simulink model "test_mdl"  (R2018a)
settings: Solver=VariableStepAuto  StartTime=0.0  StopTime=10.0  RelTol=1e-3
(part 2 of 8)

== system test_mdl/FD1_CAN_P702_GASD_MY21_DCV_V06/ABS_ESC/BrakeSnData_4 ==
  BrkTotTqRqArb_No_Cnt : Constant
  BrkTotTqRqArb_No_Cs : Constant
  BrkTot_Tq_Actl : Constant
  BrkTot_Tq_RqArb : Constant
  HsaStat_D_Actl : Constant
  VehRolComp_W_Actl : Constant
  VehVertComp_A_Actl : Constant
  bus_creator : BusCreator  Inputs=7
  port : Outport
  wires:
  bus_creator/1 -> port/1  "BrakeSnData_4"
  BrkTotTqRqArb_No_Cnt/1 -> bus_creator/1  "BrkTotTqRqArb_No_Cnt"
  BrkTotTqRqArb_No_Cs/1 -> bus_creator/2  "BrkTotTqRqArb_No_Cs"
  BrkTot_Tq_Actl/1 -> bus_creator/3  "BrkTot_Tq_Actl"
  BrkTot_Tq_RqArb/1 -> bus_creator/4  "BrkTot_Tq_RqArb"
  HsaStat_D_Actl/1 -> bus_creator/5  "HsaStat_D_Actl"
  VehRolComp_W_Actl/1 -> bus_creator/6  "VehRolComp_W_Actl"
  VehVertComp_A_Actl/1 -> bus_creator/7  "VehVertComp_A_Actl"

== system test_mdl/FD1_CAN_P702_GASD_MY21_DCV_V06/ABS_ESC/BrakeSnData_5 ==
  AwdLck_Tq_RqMn : Constant
  AwdLck_Tq_RqMx : Constant
  BrkCtrFnd_B_Stat : Constant
  DrvSte_D_Stat : Constant
  DrvSte_Tq_Rq : Constant
  EmgcyBrkLamp_D_Rq : Constant
  StopLamp_B_RqBrk : Constant
  bus_creator : BusCreator  Inputs=7
  port : Outport
  wires:
  bus_creator/1 -> port/1  "BrakeSnData_5"
  AwdLck_Tq_RqMn/1 -> bus_creator/1  "AwdLck_Tq_RqMn"
  AwdLck_Tq_RqMx/1 -> bus_creator/2  "AwdLck_Tq_RqMx"
  BrkCtrFnd_B_Stat/1 -> bus_creator/3  "BrkCtrFnd_B_Stat"
  DrvSte_D_Stat/1 -> bus_creator/4  "DrvSte_D_Stat"
  DrvSte_Tq_Rq/1 -> bus_creator/5  "DrvSte_Tq_Rq"
  EmgcyBrkLamp_D_Rq/1 -> bus_creator/6  "EmgcyBrkLamp_D_Rq"
  StopLamp_B_RqBrk/1 -> bus_creator/7  "StopLamp_B_RqBrk"

== system test_mdl/FD1_CAN_P702_GASD_MY21_DCV_V06/ABS_ESC/BrakeSnData_6 ==
  StePinOffst_An_Est : Constant
  StePinOffst_D_Stat : Constant
  StePinOffst_No_Cnt : Constant
  StePinOffst_No_Cs : Constant
  bus_creator : BusCreator  Inputs=4
  port : Outport
  wires:
  bus_creator/1 -> port/1  "BrakeSnData_6"
  StePinOffst_An_Est/1 -> bus_creator/1  "StePinOffst_An_Est"
  StePinOffst_D_Stat/1 -> bus_creator/2  "StePinOffst_D_Stat"
  StePinOffst_No_Cnt/1 -> bus_creator/3  "StePinOffst_No_Cnt"
  StePinOffst_No_Cs/1 -> bus_creator/4  "StePinOffst_No_Cs"

== system test_mdl/FD1_CAN_P702_GASD_MY21_DCV_V06/ABS_ESC/BrakeSysFeatures ==
  BrkFluidLvl_D_Stat : Constant
  LsmcBrkDecel_D_Stat : Constant
  VehStab_D_Stat : Constant
  VehVActlBrk_D_Qf : Constant
  VehVActlBrk_No_Cnt : Constant
  VehVActlBrk_No_Cs : Constant
  VehYawLin_W_Rq : Constant
  VehYawNonLin_W_Rq : Constant
  Veh_V_ActlBrk : Constant
  bus_creator : BusCreator  Inputs=9
  port : Outport
  wires:
  bus_creator/1 -> port/1  "BrakeSysFeatures"
  BrkFluidLvl_D_Stat/1 -> bus_creator/1  "BrkFluidLvl_D_Stat"
  LsmcBrkDecel_D_Stat/1 -> bus_creator/2  "LsmcBrkDecel_D_Stat"
  VehStab_D_Stat/1 -> bus_creator/3  "VehStab_D_Stat"
  VehVActlBrk_D_Qf/1 -> bus_creator/4  "VehVActlBrk_D_Qf"
  VehVActlBrk_No_Cnt/1 -> bus_creator/5  "VehVActlBrk_No_Cnt"
  VehVActlBrk_No_Cs/1 -> bus_creator/6  "VehVActlBrk_No_Cs"
  VehYawLin_W_Rq/1 -> bus_creator/7  "VehYawLin_W_Rq"
  VehYawNonLin_W_Rq/1 -> bus_creator/8  "VehYawNonLin_W_Rq"
  Veh_V_ActlBrk/1 -> bus_creator/9  "Veh_V_ActlBrk"

== system test_mdl/FD1_CAN_P702_GASD_MY21_DCV_V06/ABS_ESC/BrakeSysFeatures_2 ==
  Abs_B_Falt : Constant
  BpedMove_D_Actl : Constant
  BpedMove_No_Cnt : Constant
  BrkBstrVac_B_Rq : Constant
  BrkLamp_B_Rq : Constant
  ChimeBrk_B_Rq : Constant
  DrvAntiLckLamp_D_Rq : Constant
  DrvHdcLampInfo_D_Rq : Constant
  DrvHdcMsg_D_Rq : Constant
  DrvHdcWarnInfo_D_Rq : Constant
  DrvSlipCtlLamp_D_Rq : Constant
  DrvSlipCtlMde_D_Ind : Constant
  HILL_DESC_MC : Constant
  HdcMde_D_Actl : Constant
  HsaMde_D_Mem : Constant
  RearDiffElckrOpen_B_Rq : Constant
  RearDiffLck_Tq2_RqMx : Constant
  StabCtlBrk_B_Avail : Constant
  TCMode : Constant
  TRLR_SWAY_CONFIG_STAT : Constant
  TRLR_SWAY_EVNT_IN_PROG : Constant
  bus_creator : BusCreator  Inputs=21
  port : Outport
  wires:
  bus_creator/1 -> port/1  "BrakeSysFeatures_2"
  Abs_B_Falt/1 -> bus_creator/1  "Abs_B_Falt"
  BpedMove_D_Actl/1 -> bus_creator/2  "BpedMove_D_Actl"
  BpedMove_No_Cnt/1 -> bus_creator/3  "BpedMove_No_Cnt"
  BrkBstrVac_B_Rq/1 -> bus_creator/4  "BrkBstrVac_B_Rq"
  BrkLamp_B_Rq/1 -> bus_creator/5  "BrkLamp_B_Rq"
  ChimeBrk_B_Rq/1 -> bus_creator/6  "ChimeBrk_B_Rq"
  DrvAntiLckLamp_D_Rq/1 -> bus_creator/7  "DrvAntiLckLamp_D_Rq"
  DrvHdcLampInfo_D_Rq/1 -> bus_creator/8  "DrvHdcLampInfo_D_Rq"
  DrvHdcMsg_D_Rq/1 -> bus_creator/9  "DrvHdcMsg_D_Rq"
  DrvHdcWarnInfo_D_Rq/1 -> bus_creator/10  "DrvHdcWarnInfo_D_Rq"
  DrvSlipCtlLamp_D_Rq/1 -> bus_creator/11  "DrvSlipCtlLamp_D_Rq"
  DrvSlipCtlMde_D_Ind/1 -> bus_creator/12  "DrvSlipCtlMde_D_Ind"
  HILL_DESC_MC/1 -> bus_creator/13  "HILL_DESC_MC"
  HdcMde_D_Actl/1 -> bus_creator/14  "HdcMde_D_Actl"
  HsaMde_D_Mem/1 -> bus_creator/15  "HsaMde_D_Mem"
  RearDiffElckrOpen_B_Rq/1 -> bus_creator/16  "RearDiffElckrOpen_B_Rq"
  RearDiffLck_Tq2_RqMx/1 -> bus_creator/17  "RearDiffLck_Tq2_RqMx"
  StabCtlBrk_B_Avail/1 -> bus_creator/18  "StabCtlBrk_B_Avail"
  TCMode/1 -> bus_creator/19  "TCMode"
  TRLR_SWAY_CONFIG_STAT/1 -> bus_creator/20  "TRLR_SWAY_CONFIG_STAT"
  TRLR_SWAY_EVNT_IN_PROG/1 -> bus_creator/21  "TRLR_SWAY_EVNT_IN_PROG"

== system test_mdl/FD1_CAN_P702_GASD_MY21_DCV_V06/ABS_ESC/BrakeSysFeatures_3 ==
  AirDamUp_B_RqBrk : Constant
  ApaBrk_D_Stat : Constant
  AutoHoldMde_D_Ind : Constant
  AutoHoldMsgTxt_D_Rq : Constant
  AutoHoldSwMde_B_Ind : Constant
  BrkBstrVac_D_Stat : Constant
  CtaBrk_D_Stat : Constant
  DrvSlipCtlMdeMsg_D_Rq : Constant
  DrvSlipCtlOffLamp_D_Rq : Constant
  RbaBrk_D_Stat : Constant
  SelDrvMdeAwd_D_Rq : Constant
  SelDrvMdeChassis2_D_Rq : Constant
  SelDrvMdeChassis_D_Rq : Constant
  TrailCtlMsgTxt_D_Rq : Constant
  TrailCtl_D_Stat : Constant
  bus_creator : BusCreator  Inputs=15
  port : Outport
  wires:
  bus_creator/1 -> port/1  "BrakeSysFeatures_3"
  AirDamUp_B_RqBrk/1 -> bus_creator/1  "AirDamUp_B_RqBrk"
  ApaBrk_D_Stat/1 -> bus_creator/2  "ApaBrk_D_Stat"
  AutoHoldMde_D_Ind/1 -> bus_creator/3  "AutoHoldMde_D_Ind"
  AutoHoldMsgTxt_D_Rq/1 -> bus_creator/4  "AutoHoldMsgTxt_D_Rq"
  AutoHoldSwMde_B_Ind/1 -> bus_creator/5  "AutoHoldSwMde_B_Ind"
  BrkBstrVac_D_Stat/1 -> bus_creator/6  "BrkBstrVac_D_Stat"
  CtaBrk_D_Stat/1 -> bus_creator/7  "CtaBrk_D_Stat"
  DrvSlipCtlMdeMsg_D_Rq/1 -> bus_creator/8  "DrvSlipCtlMdeMsg_D_Rq"
  DrvSlipCtlOffLamp_D_Rq/1 -> bus_creator/9  "DrvSlipCtlOffLamp_D_Rq"
  RbaBrk_D_Stat/1 -> bus_creator/10  "RbaBrk_D_Stat"
  SelDrvMdeAwd_D_Rq/1 -> bus_creator/11  "SelDrvMdeAwd_D_Rq"
  SelDrvMdeChassis2_D_Rq/1 -> bus_creator/12  "SelDrvMdeChassis2_D_Rq"
  SelDrvMdeChassis_D_Rq/1 -> bus_creator/13  "SelDrvMdeChassis_D_Rq"
  TrailCtlMsgTxt_D_Rq/1 -> bus_creator/14  "TrailCtlMsgTxt_D_Rq"
  TrailCtl_D_Stat/1 -> bus_creator/15  "TrailCtl_D_Stat"

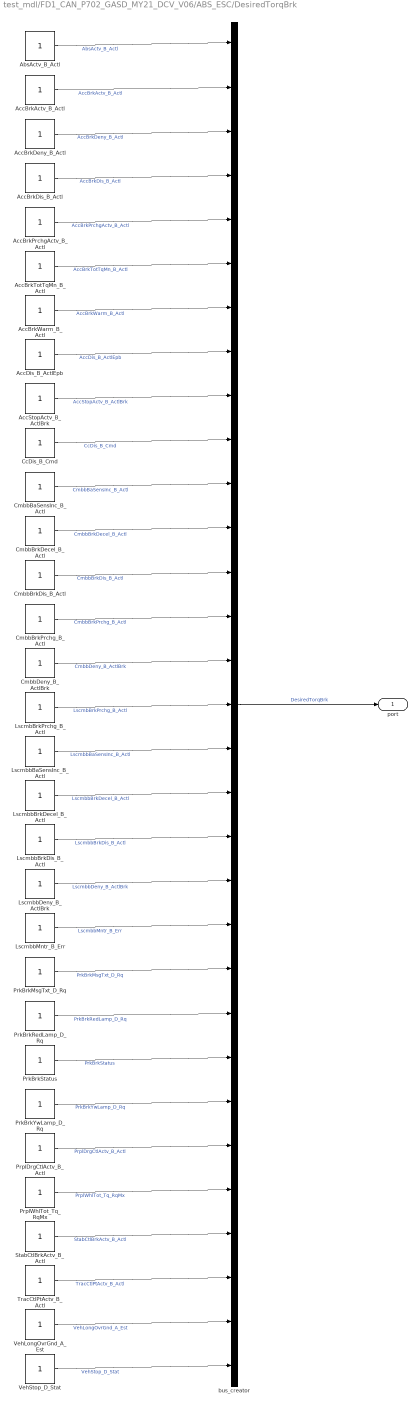
== system test_mdl/FD1_CAN_P702_GASD_MY21_DCV_V06/ABS_ESC/DesiredTorqBrk ==
  AbsActv_B_Actl : Constant
  AccBrkActv_B_Actl : Constant
  AccBrkDeny_B_Actl : Constant
  AccBrkDis_B_Actl : Constant
  AccBrkPrchgActv_B_Actl : Constant
  AccBrkTotTqMn_B_Actl : Constant
  AccBrkWarm_B_Actl : Constant
  AccDis_B_ActlEpb : Constant
  AccStopActv_B_ActlBrk : Constant
  CcDis_B_Cmd : Constant
  CmbbBaSensInc_B_Actl : Constant
  CmbbBrkDecel_B_Actl : Constant
  CmbbBrkDis_B_Actl : Constant
  CmbbBrkPrchg_B_Actl : Constant
  CmbbDeny_B_ActlBrk : Constant
  LscmbBrkPrchg_B_Actl : Constant
  LscmbbBaSensInc_B_Actl : Constant
  LscmbbBrkDecel_B_Actl : Constant
  LscmbbBrkDis_B_Actl : Constant
  LscmbbDeny_B_ActlBrk : Constant
  LscmbbMntr_B_Err : Constant
  PrkBrkMsgTxt_D_Rq : Constant
  PrkBrkRedLamp_D_Rq : Constant
  PrkBrkStatus : Constant
  PrkBrkYwLamp_D_Rq : Constant
  PrplDrgCtlActv_B_Actl : Constant
  PrplWhlTot_Tq_RqMx : Constant
  StabCtlBrkActv_B_Actl : Constant
  TracCtlPtActv_B_Actl : Constant
  VehLongOvrGnd_A_Est : Constant
  VehStop_D_Stat : Constant
  bus_creator : BusCreator  Inputs=31
  port : Outport
  wires:
  bus_creator/1 -> port/1  "DesiredTorqBrk"
  AbsActv_B_Actl/1 -> bus_creator/1  "AbsActv_B_Actl"
  AccBrkActv_B_Actl/1 -> bus_creator/2  "AccBrkActv_B_Actl"
  AccBrkDeny_B_Actl/1 -> bus_creator/3  "AccBrkDeny_B_Actl"
  AccBrkDis_B_Actl/1 -> bus_creator/4  "AccBrkDis_B_Actl"
  AccBrkPrchgActv_B_Actl/1 -> bus_creator/5  "AccBrkPrchgActv_B_Actl"
  AccBrkTotTqMn_B_Actl/1 -> bus_creator/6  "AccBrkTotTqMn_B_Actl"
  AccBrkWarm_B_Actl/1 -> bus_creator/7  "AccBrkWarm_B_Actl"
  AccDis_B_ActlEpb/1 -> bus_creator/8  "AccDis_B_ActlEpb"
  AccStopActv_B_ActlBrk/1 -> bus_creator/9  "AccStopActv_B_ActlBrk"
  CcDis_B_Cmd/1 -> bus_creator/10  "CcDis_B_Cmd"
  CmbbBaSensInc_B_Actl/1 -> bus_creator/11  "CmbbBaSensInc_B_Actl"
  CmbbBrkDecel_B_Actl/1 -> bus_creator/12  "CmbbBrkDecel_B_Actl"
  CmbbBrkDis_B_Actl/1 -> bus_creator/13  "CmbbBrkDis_B_Actl"
  CmbbBrkPrchg_B_Actl/1 -> bus_creator/14  "CmbbBrkPrchg_B_Actl"
  CmbbDeny_B_ActlBrk/1 -> bus_creator/15  "CmbbDeny_B_ActlBrk"
  LscmbBrkPrchg_B_Actl/1 -> bus_creator/16  "LscmbBrkPrchg_B_Actl"
  LscmbbBaSensInc_B_Actl/1 -> bus_creator/17  "LscmbbBaSensInc_B_Actl"
  LscmbbBrkDecel_B_Actl/1 -> bus_creator/18  "LscmbbBrkDecel_B_Actl"
  LscmbbBrkDis_B_Actl/1 -> bus_creator/19  "LscmbbBrkDis_B_Actl"
  LscmbbDeny_B_ActlBrk/1 -> bus_creator/20  "LscmbbDeny_B_ActlBrk"
  LscmbbMntr_B_Err/1 -> bus_creator/21  "LscmbbMntr_B_Err"
  PrkBrkMsgTxt_D_Rq/1 -> bus_creator/22  "PrkBrkMsgTxt_D_Rq"
  PrkBrkRedLamp_D_Rq/1 -> bus_creator/23  "PrkBrkRedLamp_D_Rq"
  PrkBrkStatus/1 -> bus_creator/24  "PrkBrkStatus"
  PrkBrkYwLamp_D_Rq/1 -> bus_creator/25  "PrkBrkYwLamp_D_Rq"
  PrplDrgCtlActv_B_Actl/1 -> bus_creator/26  "PrplDrgCtlActv_B_Actl"
  PrplWhlTot_Tq_RqMx/1 -> bus_creator/27  "PrplWhlTot_Tq_RqMx"
  StabCtlBrkActv_B_Actl/1 -> bus_creator/28  "StabCtlBrkActv_B_Actl"
  TracCtlPtActv_B_Actl/1 -> bus_creator/29  "TracCtlPtActv_B_Actl"
  VehLongOvrGnd_A_Est/1 -> bus_creator/30  "VehLongOvrGnd_A_Est"
  VehStop_D_Stat/1 -> bus_creator/31  "VehStop_D_Stat"

== system test_mdl/FD1_CAN_P702_GASD_MY21_DCV_V06/ABS_ESC/DesiredTorqBrk_2 ==
  PrplWhlTot_Tq_RqMn : Constant
  PrplWhlTqRqMn_No_Cnt : Constant
  PrplWhlTqRqMn_No_Cs : Constant
  RgenBrkDynoMde_B_Actl : Constant
  RgenTqFalt_B_Actl : Constant
  bus_creator : BusCreator  Inputs=5
  port : Outport
  wires:
  bus_creator/1 -> port/1  "DesiredTorqBrk_2"
  PrplWhlTot_Tq_RqMn/1 -> bus_creator/1  "PrplWhlTot_Tq_RqMn"
  PrplWhlTqRqMn_No_Cnt/1 -> bus_creator/2  "PrplWhlTqRqMn_No_Cnt"
  PrplWhlTqRqMn_No_Cs/1 -> bus_creator/3  "PrplWhlTqRqMn_No_Cs"
  RgenBrkDynoMde_B_Actl/1 -> bus_creator/4  "RgenBrkDynoMde_B_Actl"
  RgenTqFalt_B_Actl/1 -> bus_creator/5  "RgenTqFalt_B_Actl"

== system test_mdl/FD1_CAN_P702_GASD_MY21_DCV_V06/ABS_ESC/Global_PATS_SubTarget ==
  bus_creator : BusCreator  Inputs=2
  immoSubTarget1Cmd_T1 : Constant
  immoSubTarget1Data_T1 : Constant
  port : Outport
  wires:
  bus_creator/1 -> port/1  "Global_PATS_SubTarget"
  immoSubTarget1Cmd_T1/1 -> bus_creator/1  "immoSubTarget1Cmd_T1"
  immoSubTarget1Data_T1/1 -> bus_creator/2  "immoSubTarget1Data_T1"

== system test_mdl/FD1_CAN_P702_GASD_MY21_DCV_V06/ABS_ESC/OTAPhysABStoGWM_ECG ==
  OTAPhysABStoGWM_ECG : Constant
  bus_creator : BusCreator  Inputs=1
  port : Outport
  wires:
  bus_creator/1 -> port/1  "OTAPhysABStoGWM_ECG"
  OTAPhysABStoGWM_ECG/1 -> bus_creator/1  "OTAPhysABStoGWM_ECG"

== system test_mdl/FD1_CAN_P702_GASD_MY21_DCV_V06/ABS_ESC/PARSEDPhysABStoGWM_ECG ==
  PARSEDPhysABStoGWM_ECG : Constant
  bus_creator : BusCreator  Inputs=1
  port : Outport
  wires:
  bus_creator/1 -> port/1  "PARSEDPhysABStoGWM_ECG"
  PARSEDPhysABStoGWM_ECG/1 -> bus_creator/1  "PARSEDPhysABStoGWM_ECG"

== system test_mdl/FD1_CAN_P702_GASD_MY21_DCV_V06/ABS_ESC/PARSEDPushABStoGWM_ECG ==
  PARSEDPhysABS2toGWM_ECG : Constant
  bus_creator : BusCreator  Inputs=1
  port : Outport
  wires:
  bus_creator/1 -> port/1  "PARSEDPushABStoGWM_ECG"
  PARSEDPhysABS2toGWM_ECG/1 -> bus_creator/1  "PARSEDPhysABS2toGWM_ECG"

== system test_mdl/FD1_CAN_P702_GASD_MY21_DCV_V06/ABS_ESC/SelectDriveModeData ==
  ActvDrvMde_D2_Stat : Constant
  AutoEpbButtnOn_B_Stat : Constant
  AutoEpbDsply_D_Stat : Constant
  AutoEpbMsgTxt_D_Rq : Constant
  AwdMde_D_RqBrk : Constant
  SelDrvMdeMsgTxt_D_Rq : Constant
  SelDrvMdePos01_B_Avail : Constant
  SelDrvMdePos02_B_Avail : Constant
  SelDrvMdePos03_B_Avail : Constant
  SelDrvMdePos04_B_Avail : Constant
  SelDrvMdePos05_B_Avail : Constant
  SelDrvMdePos06_B_Avail : Constant
  SelDrvMdePos07_B_Avail : Constant
  SelDrvMdePos08_B_Avail : Constant
  SelDrvMdePos09_B_Avail : Constant
  SelDrvMdePos10_B_Avail : Constant
  SelDrvMdePos11_B_Avail : Constant
  SelDrvMdePos12_B_Avail : Constant
  SelDrvMdePt_D_Rq : Constant
  SelDrvMde_D2_Rq : Constant
  SelDrvMde_D_Stat : Constant
  bus_creator : BusCreator  Inputs=21
  port : Outport
  wires:
  bus_creator/1 -> port/1  "SelectDriveModeData"
  ActvDrvMde_D2_Stat/1 -> bus_creator/1  "ActvDrvMde_D2_Stat"
  AutoEpbButtnOn_B_Stat/1 -> bus_creator/2  "AutoEpbButtnOn_B_Stat"
  AutoEpbDsply_D_Stat/1 -> bus_creator/3  "AutoEpbDsply_D_Stat"
  AutoEpbMsgTxt_D_Rq/1 -> bus_creator/4  "AutoEpbMsgTxt_D_Rq"
  AwdMde_D_RqBrk/1 -> bus_creator/5  "AwdMde_D_RqBrk"
  SelDrvMdeMsgTxt_D_Rq/1 -> bus_creator/6  "SelDrvMdeMsgTxt_D_Rq"
  SelDrvMdePos01_B_Avail/1 -> bus_creator/7  "SelDrvMdePos01_B_Avail"
  SelDrvMdePos02_B_Avail/1 -> bus_creator/8  "SelDrvMdePos02_B_Avail"
  SelDrvMdePos03_B_Avail/1 -> bus_creator/9  "SelDrvMdePos03_B_Avail"
  SelDrvMdePos04_B_Avail/1 -> bus_creator/10  "SelDrvMdePos04_B_Avail"
  SelDrvMdePos05_B_Avail/1 -> bus_creator/11  "SelDrvMdePos05_B_Avail"
  SelDrvMdePos06_B_Avail/1 -> bus_creator/12  "SelDrvMdePos06_B_Avail"
  SelDrvMdePos07_B_Avail/1 -> bus_creator/13  "SelDrvMdePos07_B_Avail"
  SelDrvMdePos08_B_Avail/1 -> bus_creator/14  "SelDrvMdePos08_B_Avail"
  SelDrvMdePos09_B_Avail/1 -> bus_creator/15  "SelDrvMdePos09_B_Avail"
  SelDrvMdePos10_B_Avail/1 -> bus_creator/16  "SelDrvMdePos10_B_Avail"
  SelDrvMdePos11_B_Avail/1 -> bus_creator/17  "SelDrvMdePos11_B_Avail"
  SelDrvMdePos12_B_Avail/1 -> bus_creator/18  "SelDrvMdePos12_B_Avail"
  SelDrvMdePt_D_Rq/1 -> bus_creator/19  "SelDrvMdePt_D_Rq"
  SelDrvMde_D2_Rq/1 -> bus_creator/20  "SelDrvMde_D2_Rq"
  SelDrvMde_D_Stat/1 -> bus_creator/21  "SelDrvMde_D_Stat"

== system test_mdl/FD1_CAN_P702_GASD_MY21_DCV_V06/ABS_ESC/SelectDriveModeData2 ==
  SelDrvMdePos01_D_Stat : Constant
  SelDrvMdePos02_D_Stat : Constant
  SelDrvMdePos03_D_Stat : Constant
  SelDrvMdePos04_D_Stat : Constant
  SelDrvMdePos05_D_Stat : Constant
  SelDrvMdePos06_D_Stat : Constant
  SelDrvMdePos07_D_Stat : Constant
  SelDrvMdePos08_D_Stat : Constant
  SelDrvMdePos09_D_Stat : Constant
  SelDrvMdePos10_D_Stat : Constant
  SelDrvMdePos11_D_Stat : Constant
  SelDrvMdePos12_D_Stat : Constant
  bus_creator : BusCreator  Inputs=12
  port : Outport
  wires:
  bus_creator/1 -> port/1  "SelectDriveModeData2"
  SelDrvMdePos01_D_Stat/1 -> bus_creator/1  "SelDrvMdePos01_D_Stat"
  SelDrvMdePos02_D_Stat/1 -> bus_creator/2  "SelDrvMdePos02_D_Stat"
  SelDrvMdePos03_D_Stat/1 -> bus_creator/3  "SelDrvMdePos03_D_Stat"
  SelDrvMdePos04_D_Stat/1 -> bus_creator/4  "SelDrvMdePos04_D_Stat"
  SelDrvMdePos05_D_Stat/1 -> bus_creator/5  "SelDrvMdePos05_D_Stat"
  SelDrvMdePos06_D_Stat/1 -> bus_creator/6  "SelDrvMdePos06_D_Stat"
  SelDrvMdePos07_D_Stat/1 -> bus_creator/7  "SelDrvMdePos07_D_Stat"
  SelDrvMdePos08_D_Stat/1 -> bus_creator/8  "SelDrvMdePos08_D_Stat"
  SelDrvMdePos09_D_Stat/1 -> bus_creator/9  "SelDrvMdePos09_D_Stat"
  SelDrvMdePos10_D_Stat/1 -> bus_creator/10  "SelDrvMdePos10_D_Stat"
  SelDrvMdePos11_D_Stat/1 -> bus_creator/11  "SelDrvMdePos11_D_Stat"
  SelDrvMdePos12_D_Stat/1 -> bus_creator/12  "SelDrvMdePos12_D_Stat"

== system test_mdl/FD1_CAN_P702_GASD_MY21_DCV_V06/ABS_ESC/TesterPhysicalResABS ==
  TesterPhysicalResABS : Constant
  bus_creator : BusCreator  Inputs=1
  port : Outport
  wires:
  bus_creator/1 -> port/1  "TesterPhysicalResABS"
  TesterPhysicalResABS/1 -> bus_creator/1  "TesterPhysicalResABS"

== system test_mdl/FD1_CAN_P702_GASD_MY21_DCV_V06/ABS_ESC/TrailerBrakeData ==
  TrlrBrk_Pc_Rq : Constant
  VehPtch_An_Dsply : Constant
  VehRol_An_Dsply : Constant
  bus_creator : BusCreator  Inputs=3
  port : Outport
  wires:
  bus_creator/1 -> port/1  "TrailerBrakeData"
  TrlrBrk_Pc_Rq/1 -> bus_creator/1  "TrlrBrk_Pc_Rq"
  VehPtch_An_Dsply/1 -> bus_creator/2  "VehPtch_An_Dsply"
  VehRol_An_Dsply/1 -> bus_creator/3  "VehRol_An_Dsply"

== system test_mdl/FD1_CAN_P702_GASD_MY21_DCV_V06/ABS_ESC/WheelData ==
  BrkObdData_No_Actl : Constant
  BrkObdIndex_No_Actl : Constant
  WhlDirFl_D_Actl : Constant
  WhlDirFr_D_Actl : Constant
  WhlDirRl_D_Actl : Constant
  WhlDirRr_D_Actl : Constant
  WhlRotatFl_No_Cnt : Constant
  WhlRotatFr_No_Cnt : Constant
  WhlRotatRl_No_Cnt : Constant
  WhlRotatRr_No_Cnt : Constant
  bus_creator : BusCreator  Inputs=10
  port : Outport
  wires:
  bus_creator/1 -> port/1  "WheelData"
  BrkObdData_No_Actl/1 -> bus_creator/1  "BrkObdData_No_Actl"
  BrkObdIndex_No_Actl/1 -> bus_creator/2  "BrkObdIndex_No_Actl"
  WhlDirFl_D_Actl/1 -> bus_creator/3  "WhlDirFl_D_Actl"
  WhlDirFr_D_Actl/1 -> bus_creator/4  "WhlDirFr_D_Actl"
  WhlDirRl_D_Actl/1 -> bus_creator/5  "WhlDirRl_D_Actl"
  WhlDirRr_D_Actl/1 -> bus_creator/6  "WhlDirRr_D_Actl"
  WhlRotatFl_No_Cnt/1 -> bus_creator/7  "WhlRotatFl_No_Cnt"
  WhlRotatFr_No_Cnt/1 -> bus_creator/8  "WhlRotatFr_No_Cnt"
  WhlRotatRl_No_Cnt/1 -> bus_creator/9  "WhlRotatRl_No_Cnt"
  WhlRotatRr_No_Cnt/1 -> bus_creator/10  "WhlRotatRr_No_Cnt"

== system test_mdl/FD1_CAN_P702_GASD_MY21_DCV_V06/ABS_ESC/WheelSpeed ==
  WhlFl_W_Meas : Constant
  WhlFr_W_Meas : Constant
  WhlRl_W_Meas : Constant
  WhlRr_W_Meas : Constant
  bus_creator : BusCreator  Inputs=4
  port : Outport
  wires:
  bus_creator/1 -> port/1  "WheelSpeed"
  WhlFl_W_Meas/1 -> bus_creator/1  "WhlFl_W_Meas"
  WhlFr_W_Meas/1 -> bus_creator/2  "WhlFr_W_Meas"
  WhlRl_W_Meas/1 -> bus_creator/3  "WhlRl_W_Meas"
  WhlRr_W_Meas/1 -> bus_creator/4  "WhlRr_W_Meas"

== system test_mdl/FD1_CAN_P702_GASD_MY21_DCV_V06/CMR_DSMC/CMR_DSMC_AutoSar_NetwrkMgt ==
  CMR_DSMC_AutoSarNMControl : Constant
  CMR_DSMC_AutoSarNMNodeId : Constant
  CMR_DSMC_AutoSarNMReserve2 : Constant
  CMR_DSMC_AutoSarNMReserve3 : Constant
  CMR_DSMC_AutoSarNMReserve4 : Constant
  CMR_DSMC_AutoSarNMReserved : Constant
  CMR_DSMC_GWNMProxY : Constant
  CMR_DSMC_GWOnBoardTester : Constant
  bus_creator : BusCreator  Inputs=8
  port : Outport
  wires:
  bus_creator/1 -> port/1  "CMR_DSMC_AutoSar_NetwrkMgt"
  CMR_DSMC_AutoSarNMControl/1 -> bus_creator/1  "CMR_DSMC_AutoSarNMControl"
  CMR_DSMC_AutoSarNMNodeId/1 -> bus_creator/2  "CMR_DSMC_AutoSarNMNodeId"
  CMR_DSMC_AutoSarNMReserve2/1 -> bus_creator/3  "CMR_DSMC_AutoSarNMReserve2"
  CMR_DSMC_AutoSarNMReserve3/1 -> bus_creator/4  "CMR_DSMC_AutoSarNMReserve3"
  CMR_DSMC_AutoSarNMReserve4/1 -> bus_creator/5  "CMR_DSMC_AutoSarNMReserve4"
  CMR_DSMC_AutoSarNMReserved/1 -> bus_creator/6  "CMR_DSMC_AutoSarNMReserved"
  CMR_DSMC_GWNMProxY/1 -> bus_creator/7  "CMR_DSMC_GWNMProxY"
  CMR_DSMC_GWOnBoardTester/1 -> bus_creator/8  "CMR_DSMC_GWOnBoardTester"

== system test_mdl/FD1_CAN_P702_GASD_MY21_DCV_V06/CMR_DSMC/DrvStatMonData ==
  DrvAlertSt_D_Stat : Constant
  DrvAttentZone_D_Stat : Constant
  DrvCamDrvIR_D_Stat : Constant
  DrvCamPassIR_D_Stat : Constant
  DrvCamera_D_Stat : Constant
  DrvEngLvlConfid_D_Stat : Constant
  DrvEngageLevel_D_Stat : Constant
  DrvEngageLevel_No_Cnt : Constant
  DrvEngageLevel_No_Cs : Constant
  DrvImpLvlConfid_D_Stat : Constant
  DrvImpairLvl_D_Stat : Constant
  bus_creator : BusCreator  Inputs=11
  port : Outport
  wires:
  bus_creator/1 -> port/1  "DrvStatMonData"
  DrvAlertSt_D_Stat/1 -> bus_creator/1  "DrvAlertSt_D_Stat"
  DrvAttentZone_D_Stat/1 -> bus_creator/2  "DrvAttentZone_D_Stat"
  DrvCamDrvIR_D_Stat/1 -> bus_creator/3  "DrvCamDrvIR_D_Stat"
  DrvCamPassIR_D_Stat/1 -> bus_creator/4  "DrvCamPassIR_D_Stat"
  DrvCamera_D_Stat/1 -> bus_creator/5  "DrvCamera_D_Stat"
  DrvEngLvlConfid_D_Stat/1 -> bus_creator/6  "DrvEngLvlConfid_D_Stat"
  DrvEngageLevel_D_Stat/1 -> bus_creator/7  "DrvEngageLevel_D_Stat"
  DrvEngageLevel_No_Cnt/1 -> bus_creator/8  "DrvEngageLevel_No_Cnt"
  DrvEngageLevel_No_Cs/1 -> bus_creator/9  "DrvEngageLevel_No_Cs"
  DrvImpLvlConfid_D_Stat/1 -> bus_creator/10  "DrvImpLvlConfid_D_Stat"
  DrvImpairLvl_D_Stat/1 -> bus_creator/11  "DrvImpairLvl_D_Stat"

== system test_mdl/FD1_CAN_P702_GASD_MY21_DCV_V06/CMR_DSMC/TesterPhysicalResCMR_DSMC ==
  TesterPhysicalResCMR_DSMC : Constant
  bus_creator : BusCreator  Inputs=1
  port : Outport
  wires:
  bus_creator/1 -> port/1  "TesterPhysicalResCMR_DSMC"
  TesterPhysicalResCMR_DSMC/1 -> bus_creator/1  "TesterPhysicalResCMR_DSMC"

== system test_mdl/FD1_CAN_P702_GASD_MY21_DCV_V06/ECM_Diesel/CGEA_Urea_Strategy ==
  DieslPrtcWarn_D_Rq : Constant
  UreaLvlQlty_D_RqDsply : Constant
  UreaLvlTxtWarn_D_Rq : Constant
  UreaLvlTxt_D_RqDsply : Constant
  UreaLvl_Pc_Actl : Constant
  UreaQltyFlg_B_RqDsply : Constant
  UreaQltySysWarn_D_Rq : Constant
  UreaQltySys_D_RqDsply : Constant
  VehUreaRnge2_L_DsplyMx : Constant
  VehUreaWarn_V_DsplyMx : Constant
  bus_creator : BusCreator  Inputs=10
  port : Outport
  wires:
  bus_creator/1 -> port/1  "CGEA_Urea_Strategy"
  DieslPrtcWarn_D_Rq/1 -> bus_creator/1  "DieslPrtcWarn_D_Rq"
  UreaLvlQlty_D_RqDsply/1 -> bus_creator/2  "UreaLvlQlty_D_RqDsply"
  UreaLvlTxtWarn_D_Rq/1 -> bus_creator/3  "UreaLvlTxtWarn_D_Rq"
  UreaLvlTxt_D_RqDsply/1 -> bus_creator/4  "UreaLvlTxt_D_RqDsply"
  UreaLvl_Pc_Actl/1 -> bus_creator/5  "UreaLvl_Pc_Actl"
  UreaQltyFlg_B_RqDsply/1 -> bus_creator/6  "UreaQltyFlg_B_RqDsply"
  UreaQltySysWarn_D_Rq/1 -> bus_creator/7  "UreaQltySysWarn_D_Rq"
  UreaQltySys_D_RqDsply/1 -> bus_creator/8  "UreaQltySys_D_RqDsply"
  VehUreaRnge2_L_DsplyMx/1 -> bus_creator/9  "VehUreaRnge2_L_DsplyMx"
  VehUreaWarn_V_DsplyMx/1 -> bus_creator/10  "VehUreaWarn_V_DsplyMx"

== system test_mdl/FD1_CAN_P702_GASD_MY21_DCV_V06/ECM_Diesel/EffDrvModeData ==
  EdmCmplnc_B_Dsply : Constant
  EdmCmplnc_Pc_Dsply : Constant
  EdmCurrent_Fe_Dsply : Constant
  EdmLamp_D_Dsply : Constant
  EdmMsgTxt_D_Rq : Constant
  EdmPrev_Fe_Dsply : Constant
  EdmSailMdeOn_B_Stat : Constant
  EdmVeh_V_Dsply : Constant
  bus_creator : BusCreator  Inputs=8
  port : Outport
  wires:
  bus_creator/1 -> port/1  "EffDrvModeData"
  EdmCmplnc_B_Dsply/1 -> bus_creator/1  "EdmCmplnc_B_Dsply"
  EdmCmplnc_Pc_Dsply/1 -> bus_creator/2  "EdmCmplnc_Pc_Dsply"
  EdmCurrent_Fe_Dsply/1 -> bus_creator/3  "EdmCurrent_Fe_Dsply"
  EdmLamp_D_Dsply/1 -> bus_creator/4  "EdmLamp_D_Dsply"
  EdmMsgTxt_D_Rq/1 -> bus_creator/5  "EdmMsgTxt_D_Rq"
  EdmPrev_Fe_Dsply/1 -> bus_creator/6  "EdmPrev_Fe_Dsply"
  EdmSailMdeOn_B_Stat/1 -> bus_creator/7  "EdmSailMdeOn_B_Stat"
  EdmVeh_V_Dsply/1 -> bus_creator/8  "EdmVeh_V_Dsply"

== system test_mdl/FD1_CAN_P702_GASD_MY21_DCV_V06/ECM_Diesel/EngBrakeData ==
  AccEngStat_D_Actl : Constant
  AccStopMde_D_Rq : Constant
  BPedDrvAppl_D_QF : Constant
  BpedDrvAppl_D_Actl : Constant
  CcMde_D_Actl : Constant
  CcOvrrdActv_B_Actl : Constant
  CcStat_D_Actl : Constant
  CmbbDeny_B_ActlPrpl : Constant
  CmbbEngTqMn_B_Actl : Constant
  EngAout_N_MnAllw : Constant
  PrplTqMnSat_B_Actl : Constant
  Veh_V_DsplyCcSet : Constant
  bus_creator : BusCreator  Inputs=12
  port : Outport
  wires:
  bus_creator/1 -> port/1  "EngBrakeData"
  AccEngStat_D_Actl/1 -> bus_creator/1  "AccEngStat_D_Actl"
  AccStopMde_D_Rq/1 -> bus_creator/2  "AccStopMde_D_Rq"
  BPedDrvAppl_D_QF/1 -> bus_creator/3  "BPedDrvAppl_D_QF"
  BpedDrvAppl_D_Actl/1 -> bus_creator/4  "BpedDrvAppl_D_Actl"
  CcMde_D_Actl/1 -> bus_creator/5  "CcMde_D_Actl"
  CcOvrrdActv_B_Actl/1 -> bus_creator/6  "CcOvrrdActv_B_Actl"
  CcStat_D_Actl/1 -> bus_creator/7  "CcStat_D_Actl"
  CmbbDeny_B_ActlPrpl/1 -> bus_creator/8  "CmbbDeny_B_ActlPrpl"
  CmbbEngTqMn_B_Actl/1 -> bus_creator/9  "CmbbEngTqMn_B_Actl"
  EngAout_N_MnAllw/1 -> bus_creator/10  "EngAout_N_MnAllw"
  PrplTqMnSat_B_Actl/1 -> bus_creator/11  "PrplTqMnSat_B_Actl"
  Veh_V_DsplyCcSet/1 -> bus_creator/12  "Veh_V_DsplyCcSet"

== system test_mdl/FD1_CAN_P702_GASD_MY21_DCV_V06/ECM_Diesel/EngVehicleSpThrottle ==
  ApedPosPcActl_D_Qf : Constant
  ApedPosPcActl_No_Cnt : Constant
  ApedPosPcActl_No_Cs : Constant
  ApedPos_PcRate_ActlArb : Constant
  ApedPos_Pc_ActlArb : Constant
  EngAout3_N_Actl : Constant
  EngAoutNActl_D_QF : Constant
  EngAout_N_Actl : Constant
  bus_creator : BusCreator  Inputs=8
  port : Outport
  wires:
  bus_creator/1 -> port/1  "EngVehicleSpThrottle"
  ApedPosPcActl_D_Qf/1 -> bus_creator/1  "ApedPosPcActl_D_Qf"
  ApedPosPcActl_No_Cnt/1 -> bus_creator/2  "ApedPosPcActl_No_Cnt"
  ApedPosPcActl_No_Cs/1 -> bus_creator/3  "ApedPosPcActl_No_Cs"
  ApedPos_PcRate_ActlArb/1 -> bus_creator/4  "ApedPos_PcRate_ActlArb"
  ApedPos_Pc_ActlArb/1 -> bus_creator/5  "ApedPos_Pc_ActlArb"
  EngAout3_N_Actl/1 -> bus_creator/6  "EngAout3_N_Actl"
  EngAoutNActl_D_QF/1 -> bus_creator/7  "EngAoutNActl_D_QF"
  EngAout_N_Actl/1 -> bus_creator/8  "EngAout_N_Actl"

== system test_mdl/FD1_CAN_P702_GASD_MY21_DCV_V06/ECM_Diesel/EngVehicleSpThrottle2 ==
  GearRvrse_D_Actl : Constant
  StrtrMtrCtlMsgTxt_D2_Rq : Constant
  StrtrMtrCtlMsgTxt_D_Rq : Constant
  StrtrMtrDlyStrt_B_Stat : Constant
  VehVActlEng_D_Qf : Constant
  VehVActlEng_No_Cnt : Constant
  VehVActlEng_No_Cs : Constant
  VehVTrlrAid_B_Avail : Constant
  Veh_V_ActlEng : Constant
  Veh_V_RqCcSet : Constant
  bus_creator : BusCreator  Inputs=10
  port : Outport
  wires:
  bus_creator/1 -> port/1  "EngVehicleSpThrottle2"
  GearRvrse_D_Actl/1 -> bus_creator/1  "GearRvrse_D_Actl"
  StrtrMtrCtlMsgTxt_D2_Rq/1 -> bus_creator/2  "StrtrMtrCtlMsgTxt_D2_Rq"
  StrtrMtrCtlMsgTxt_D_Rq/1 -> bus_creator/3  "StrtrMtrCtlMsgTxt_D_Rq"
  StrtrMtrDlyStrt_B_Stat/1 -> bus_creator/4  "StrtrMtrDlyStrt_B_Stat"
  VehVActlEng_D_Qf/1 -> bus_creator/5  "VehVActlEng_D_Qf"
  VehVActlEng_No_Cnt/1 -> bus_creator/6  "VehVActlEng_No_Cnt"
  VehVActlEng_No_Cs/1 -> bus_creator/7  "VehVActlEng_No_Cs"
  VehVTrlrAid_B_Avail/1 -> bus_creator/8  "VehVTrlrAid_B_Avail"
  Veh_V_ActlEng/1 -> bus_creator/9  "Veh_V_ActlEng"
  Veh_V_RqCcSet/1 -> bus_creator/10  "Veh_V_RqCcSet"

== system test_mdl/FD1_CAN_P702_GASD_MY21_DCV_V06/ECM_Diesel/EngineClimateData ==
  AirAmbTe_D_Qf : Constant
  AirAmb_P_Actl : Constant
  AirAmb_Te_Actl : Constant
  AirAmb_Te_ActlFilt : Constant
  AslChime_B_Rq : Constant
  AslIconDsply_D_Rq : Constant
  DynoMde_B_Cmd : Constant
  EcssLamp_D_RqDsply : Constant
  EngAout_Aa_Actl : Constant
  GasPrtc_D_RqDsply : Constant
  HvacHtrCore2_Te_Actl : Constant
  bus_creator : BusCreator  Inputs=11
  port : Outport
  wires:
  bus_creator/1 -> port/1  "EngineClimateData"
  AirAmbTe_D_Qf/1 -> bus_creator/1  "AirAmbTe_D_Qf"
  AirAmb_P_Actl/1 -> bus_creator/2  "AirAmb_P_Actl"
  AirAmb_Te_Actl/1 -> bus_creator/3  "AirAmb_Te_Actl"
  AirAmb_Te_ActlFilt/1 -> bus_creator/4  "AirAmb_Te_ActlFilt"
  AslChime_B_Rq/1 -> bus_creator/5  "AslChime_B_Rq"
  AslIconDsply_D_Rq/1 -> bus_creator/6  "AslIconDsply_D_Rq"
  DynoMde_B_Cmd/1 -> bus_creator/7  "DynoMde_B_Cmd"
  EcssLamp_D_RqDsply/1 -> bus_creator/8  "EcssLamp_D_RqDsply"
  EngAout_Aa_Actl/1 -> bus_creator/9  "EngAout_Aa_Actl"
  GasPrtc_D_RqDsply/1 -> bus_creator/10  "GasPrtc_D_RqDsply"
  HvacHtrCore2_Te_Actl/1 -> bus_creator/11  "HvacHtrCore2_Te_Actl"

== system test_mdl/FD1_CAN_P702_GASD_MY21_DCV_V06/ECM_Diesel/EngineData_10 ==
  AccFllwMdeActv_B_Actl : Constant
  AutoRgenTxt_B_RqDsply : Constant
  DieslMsgTxt_D_Rq : Constant
  EngPtoMde_D_Actl : Constant
  ManRgenSoot_Pc_RqDsply : Constant
  ManRgenTxt_D_RqDsply : Constant
  bus_creator : BusCreator  Inputs=6
  port : Outport
  wires:
  bus_creator/1 -> port/1  "EngineData_10"
  AccFllwMdeActv_B_Actl/1 -> bus_creator/1  "AccFllwMdeActv_B_Actl"
  AutoRgenTxt_B_RqDsply/1 -> bus_creator/2  "AutoRgenTxt_B_RqDsply"
  DieslMsgTxt_D_Rq/1 -> bus_creator/3  "DieslMsgTxt_D_Rq"
  EngPtoMde_D_Actl/1 -> bus_creator/4  "EngPtoMde_D_Actl"
  ManRgenSoot_Pc_RqDsply/1 -> bus_creator/5  "ManRgenSoot_Pc_RqDsply"
  ManRgenTxt_D_RqDsply/1 -> bus_creator/6  "ManRgenTxt_D_RqDsply"

== system test_mdl/FD1_CAN_P702_GASD_MY21_DCV_V06/ECM_Diesel/EngineData_11 ==
  DieslPrtc2_D_RqDsply : Constant
  DieslPrtcRgen_D_Actl : Constant
  EngExhOvrTe_B_RqDsply : Constant
  EngTeColdPrtct_D_Stats : Constant
  bus_creator : BusCreator  Inputs=4
  port : Outport
  wires:
  bus_creator/1 -> port/1  "EngineData_11"
  DieslPrtc2_D_RqDsply/1 -> bus_creator/1  "DieslPrtc2_D_RqDsply"
  DieslPrtcRgen_D_Actl/1 -> bus_creator/2  "DieslPrtcRgen_D_Actl"
  EngExhOvrTe_B_RqDsply/1 -> bus_creator/3  "EngExhOvrTe_B_RqDsply"
  EngTeColdPrtct_D_Stats/1 -> bus_creator/4  "EngTeColdPrtct_D_Stats"

== system test_mdl/FD1_CAN_P702_GASD_MY21_DCV_V06/ECM_Diesel/EngineData_16 ==
  EngAout_N_MxAllw : Constant
  EngExhBrkAutoLamp_B_Rq : Constant
  EngExhBrkMde_D_Actl : Constant
  EngExhBrkOnLamp_B_Rq : Constant
  EngOilLvlWarn_D_Rq1 : Constant
  bus_creator : BusCreator  Inputs=5
  port : Outport
  wires:
  bus_creator/1 -> port/1  "EngineData_16"
  EngAout_N_MxAllw/1 -> bus_creator/1  "EngAout_N_MxAllw"
  EngExhBrkAutoLamp_B_Rq/1 -> bus_creator/2  "EngExhBrkAutoLamp_B_Rq"
  EngExhBrkMde_D_Actl/1 -> bus_creator/3  "EngExhBrkMde_D_Actl"
  EngExhBrkOnLamp_B_Rq/1 -> bus_creator/4  "EngExhBrkOnLamp_B_Rq"
  EngOilLvlWarn_D_Rq1/1 -> bus_creator/5  "EngOilLvlWarn_D_Rq1"

== system test_mdl/FD1_CAN_P702_GASD_MY21_DCV_V06/ECM_Diesel/EngineData_17 ==
  DistToNextOilChange : Constant
  EngOilLife_T_Actl : Constant
  EngOilSrvcMsgTxt_D_Rq : Constant
  GlowIndication : Constant
  RunDryPrevent_B_Stat : Constant
  WaterInFuel : Constant
  bus_creator : BusCreator  Inputs=6
  port : Outport
  wires:
  bus_creator/1 -> port/1  "EngineData_17"
  DistToNextOilChange/1 -> bus_creator/1  "DistToNextOilChange"
  EngOilLife_T_Actl/1 -> bus_creator/2  "EngOilLife_T_Actl"
  EngOilSrvcMsgTxt_D_Rq/1 -> bus_creator/3  "EngOilSrvcMsgTxt_D_Rq"
  GlowIndication/1 -> bus_creator/4  "GlowIndication"
  RunDryPrevent_B_Stat/1 -> bus_creator/5  "RunDryPrevent_B_Stat"
  WaterInFuel/1 -> bus_creator/6  "WaterInFuel"

== system test_mdl/FD1_CAN_P702_GASD_MY21_DCV_V06/ECM_Diesel/EngineData_6 ==
  EngClntTe_D_Qf : Constant
  EngClnt_Te_Actl : Constant
  EngGoutLss_Tq_Est : Constant
  EngOil_Te_Actl : Constant
  EngOvrhtMitgActv_D_Ind : Constant
  bus_creator : BusCreator  Inputs=5
  port : Outport
  wires:
  bus_creator/1 -> port/1  "EngineData_6"
  EngClntTe_D_Qf/1 -> bus_creator/1  "EngClntTe_D_Qf"
  EngClnt_Te_Actl/1 -> bus_creator/2  "EngClnt_Te_Actl"
  EngGoutLss_Tq_Est/1 -> bus_creator/3  "EngGoutLss_Tq_Est"
  EngOil_Te_Actl/1 -> bus_creator/4  "EngOil_Te_Actl"
  EngOvrhtMitgActv_D_Ind/1 -> bus_creator/5  "EngOvrhtMitgActv_D_Ind"

== system test_mdl/FD1_CAN_P702_GASD_MY21_DCV_V06/ECM_Diesel/EngineData_7 ==
  AirCondClutch_B_Stats : Constant
  AirCondRec_B_Rq : Constant
  EngOilLife_Pc_Actl : Constant
  EngSrvcRqd_B_Rq : Constant
  FuelFillInlet_B_Dsply : Constant
  FuelFilterLamp_B_Dsply : Constant
  FuelFlw_Vl_Dsply : Constant
  HvacAirFullOut_B_Rq : Constant
  OdoCount : Constant
  bus_creator : BusCreator  Inputs=9
  port : Outport
  wires:
  bus_creator/1 -> port/1  "EngineData_7"
  AirCondClutch_B_Stats/1 -> bus_creator/1  "AirCondClutch_B_Stats"
  AirCondRec_B_Rq/1 -> bus_creator/2  "AirCondRec_B_Rq"
  EngOilLife_Pc_Actl/1 -> bus_creator/3  "EngOilLife_Pc_Actl"
  EngSrvcRqd_B_Rq/1 -> bus_creator/4  "EngSrvcRqd_B_Rq"
  FuelFillInlet_B_Dsply/1 -> bus_creator/5  "FuelFillInlet_B_Dsply"
  FuelFilterLamp_B_Dsply/1 -> bus_creator/6  "FuelFilterLamp_B_Dsply"
  FuelFlw_Vl_Dsply/1 -> bus_creator/7  "FuelFlw_Vl_Dsply"
  HvacAirFullOut_B_Rq/1 -> bus_creator/8  "HvacAirFullOut_B_Rq"
  OdoCount/1 -> bus_creator/9  "OdoCount"

== system test_mdl/FD1_CAN_P702_GASD_MY21_DCV_V06/ECM_Diesel/Engine_Clutch_Data ==
  CluPdlPosPcMeas_D_Qf : Constant
  CluPdlPos_Pc_Meas : Constant
  CluPdl_PcRate_Actl : Constant
  EngAoutIdl_N_Ntrl : Constant
  EngAout_N_Dsply : Constant
  bus_creator : BusCreator  Inputs=5
  port : Outport
  wires:
  bus_creator/1 -> port/1  "Engine_Clutch_Data"
  CluPdlPosPcMeas_D_Qf/1 -> bus_creator/1  "CluPdlPosPcMeas_D_Qf"
  CluPdlPos_Pc_Meas/1 -> bus_creator/2  "CluPdlPos_Pc_Meas"
  CluPdl_PcRate_Actl/1 -> bus_creator/3  "CluPdl_PcRate_Actl"
  EngAoutIdl_N_Ntrl/1 -> bus_creator/4  "EngAoutIdl_N_Ntrl"
  EngAout_N_Dsply/1 -> bus_creator/5  "EngAout_N_Dsply"

== system test_mdl/FD1_CAN_P702_GASD_MY21_DCV_V06/ECM_Diesel/Engine_Data_18 ==
  EngAirFiltMsgTxt_D_Rq : Constant
  UreaMnAdd_L2_Actl : Constant
  UreaMxAdd_L2_Actl : Constant
  VehUreaRnge3_L_DsplyMx : Constant
  WaterInFuel_B_Falt : Constant
  bus_creator : BusCreator  Inputs=5
  port : Outport
  wires:
  bus_creator/1 -> port/1  "Engine_Data_18"
  EngAirFiltMsgTxt_D_Rq/1 -> bus_creator/1  "EngAirFiltMsgTxt_D_Rq"
  UreaMnAdd_L2_Actl/1 -> bus_creator/2  "UreaMnAdd_L2_Actl"
  UreaMxAdd_L2_Actl/1 -> bus_creator/3  "UreaMxAdd_L2_Actl"
  VehUreaRnge3_L_DsplyMx/1 -> bus_creator/4  "VehUreaRnge3_L_DsplyMx"
  WaterInFuel_B_Falt/1 -> bus_creator/5  "WaterInFuel_B_Falt"

== system test_mdl/FD1_CAN_P702_GASD_MY21_DCV_V06/ECM_Diesel/Global_PATS_TargetInfo ==
  bus_creator : BusCreator  Inputs=3
  immoTarget1Cmd : Constant
  immoTarget1Data : Constant
  immoTarget1Status : Constant
  port : Outport
  wires:
  bus_creator/1 -> port/1  "Global_PATS_TargetInfo"
  immoTarget1Cmd/1 -> bus_creator/1  "immoTarget1Cmd"
  immoTarget1Data/1 -> bus_creator/2  "immoTarget1Data"
  immoTarget1Status/1 -> bus_creator/3  "immoTarget1Status"

== system test_mdl/FD1_CAN_P702_GASD_MY21_DCV_V06/ECM_Diesel/Low_Voltage_Power_Data_FD1 ==
  PwSrcULoComm_B_Falt : Constant
  PwSrcULoDcnnt_B_Stat : Constant
  PwSrcULoFalt_D_Stat : Constant
  PwSrcULoOvrTe_B_Actl : Constant
  PwSrcULo_I_Actl : Constant
  PwSrcULo_I_Mx : Constant
  PwSrcULo_Pc_Mx : Constant
  ULoRgenTestMde_B_Stat : Constant
  bus_creator : BusCreator  Inputs=8
  port : Outport
  wires:
  bus_creator/1 -> port/1  "Low_Voltage_Power_Data_FD1"
  PwSrcULoComm_B_Falt/1 -> bus_creator/1  "PwSrcULoComm_B_Falt"
  PwSrcULoDcnnt_B_Stat/1 -> bus_creator/2  "PwSrcULoDcnnt_B_Stat"
  PwSrcULoFalt_D_Stat/1 -> bus_creator/3  "PwSrcULoFalt_D_Stat"
  PwSrcULoOvrTe_B_Actl/1 -> bus_creator/4  "PwSrcULoOvrTe_B_Actl"
  PwSrcULo_I_Actl/1 -> bus_creator/5  "PwSrcULo_I_Actl"
  PwSrcULo_I_Mx/1 -> bus_creator/6  "PwSrcULo_I_Mx"
  PwSrcULo_Pc_Mx/1 -> bus_creator/7  "PwSrcULo_Pc_Mx"
  ULoRgenTestMde_B_Stat/1 -> bus_creator/8  "ULoRgenTestMde_B_Stat"

== system test_mdl/FD1_CAN_P702_GASD_MY21_DCV_V06/ECM_Diesel/OTAPhysPCMtoGWM_ECG ==
  OTAPhysPCMtoGWM_ECG : Constant
  bus_creator : BusCreator  Inputs=1
  port : Outport
  wires:
  bus_creator/1 -> port/1  "OTAPhysPCMtoGWM_ECG"
  OTAPhysPCMtoGWM_ECG/1 -> bus_creator/1  "OTAPhysPCMtoGWM_ECG"

== system test_mdl/FD1_CAN_P702_GASD_MY21_DCV_V06/ECM_Diesel/PARSEDPhysPCMtoGWM_ECG ==
  PARSEDPhysPCMtoGWM_ECG : Constant
  bus_creator : BusCreator  Inputs=1
  port : Outport
  wires:
  bus_creator/1 -> port/1  "PARSEDPhysPCMtoGWM_ECG"
  PARSEDPhysPCMtoGWM_ECG/1 -> bus_creator/1  "PARSEDPhysPCMtoGWM_ECG"

== system test_mdl/FD1_CAN_P702_GASD_MY21_DCV_V06/ECM_Diesel/PARSEDPushPCMtoGWM_ECG ==
  PARSEDPushPCMtoGWM_ECG : Constant
  bus_creator : BusCreator  Inputs=1
  port : Outport
  wires:
  bus_creator/1 -> port/1  "PARSEDPushPCMtoGWM_ECG"
  PARSEDPushPCMtoGWM_ECG/1 -> bus_creator/1  "PARSEDPushPCMtoGWM_ECG"

== system test_mdl/FD1_CAN_P702_GASD_MY21_DCV_V06/ECM_Diesel/PCM_AutoSar_NetworkMgmt ==
  PCM_AutoSarNMControl : Constant
  PCM_AutoSarNMNodeId : Constant
  PCM_AutoSarNMReserved{1..4} (4 alike) : Constant
  PCM_GWNMProxy : Constant
  PCM_GWOnBoardTester : Constant
  bus_creator : BusCreator  Inputs=8
  port : Outport
  wires:
  bus_creator/1 -> port/1  "PCM_AutoSar_NetworkMgmt"
  PCM_AutoSarNMControl/1 -> bus_creator/1  "PCM_AutoSarNMControl"
  PCM_AutoSarNMNodeId/1 -> bus_creator/2  "PCM_AutoSarNMNodeId"
  PCM_AutoSarNMReserved1/1 -> bus_creator/3  "PCM_AutoSarNMReserved1"
  PCM_AutoSarNMReserved2/1 -> bus_creator/4  "PCM_AutoSarNMReserved2"
  PCM_AutoSarNMReserved3/1 -> bus_creator/5  "PCM_AutoSarNMReserved3"
  PCM_AutoSarNMReserved4/1 -> bus_creator/6  "PCM_AutoSarNMReserved4"
  PCM_GWNMProxy/1 -> bus_creator/7  "PCM_GWNMProxy"
  PCM_GWOnBoardTester/1 -> bus_creator/8  "PCM_GWOnBoardTester"

== system test_mdl/FD1_CAN_P702_GASD_MY21_DCV_V06/ECM_Diesel/PCM_Rapid_Data_Response_1 ==
  UUDTPCMResponse1 : Constant
  bus_creator : BusCreator  Inputs=1
  port : Outport
  wires:
  bus_creator/1 -> port/1  "PCM_Rapid_Data_Response_1"
  UUDTPCMResponse1/1 -> bus_creator/1  "UUDTPCMResponse1"

== system test_mdl/FD1_CAN_P702_GASD_MY21_DCV_V06/ECM_Diesel/PCM_Rapid_Data_Response_2 ==
  UUDTPCMResponse2 : Constant
  bus_creator : BusCreator  Inputs=1
  port : Outport
  wires:
  bus_creator/1 -> port/1  "PCM_Rapid_Data_Response_2"
  UUDTPCMResponse2/1 -> bus_creator/1  "UUDTPCMResponse2"

== system test_mdl/FD1_CAN_P702_GASD_MY21_DCV_V06/ECM_Diesel/PowertrainData_1 ==
  AirCondFluidHi_P_Actl : Constant
  CoolantFanStepAct : Constant
  ECMMILRequest : Constant
  EngIdlShutDown_D_Stat : Constant
  EngIdlShutDwnTxt_D_Rq : Constant
  FUEL_ALCOHOL_PERCNT : Constant
  FohEng_D_Rq : Constant
  OilPressureWarning : Constant
  TrnTotLss_Tq_Est : Constant
  TrnTotTq_Rt_Est : Constant
  VehVLimActv_B_Actl : Constant
  VehVLimStat_D_Actl : Constant
  bus_creator : BusCreator  Inputs=12
  port : Outport
  wires:
  bus_creator/1 -> port/1  "PowertrainData_1"
  AirCondFluidHi_P_Actl/1 -> bus_creator/1  "AirCondFluidHi_P_Actl"
  CoolantFanStepAct/1 -> bus_creator/2  "CoolantFanStepAct"
  ECMMILRequest/1 -> bus_creator/3  "ECMMILRequest"
  EngIdlShutDown_D_Stat/1 -> bus_creator/4  "EngIdlShutDown_D_Stat"
  EngIdlShutDwnTxt_D_Rq/1 -> bus_creator/5  "EngIdlShutDwnTxt_D_Rq"
  FUEL_ALCOHOL_PERCNT/1 -> bus_creator/6  "FUEL_ALCOHOL_PERCNT"
  FohEng_D_Rq/1 -> bus_creator/7  "FohEng_D_Rq"
  OilPressureWarning/1 -> bus_creator/8  "OilPressureWarning"
  TrnTotLss_Tq_Est/1 -> bus_creator/9  "TrnTotLss_Tq_Est"
  TrnTotTq_Rt_Est/1 -> bus_creator/10  "TrnTotTq_Rt_Est"
  VehVLimActv_B_Actl/1 -> bus_creator/11  "VehVLimActv_B_Actl"
  VehVLimStat_D_Actl/1 -> bus_creator/12  "VehVLimStat_D_Actl"

== system test_mdl/FD1_CAN_P702_GASD_MY21_DCV_V06/ECM_Diesel/PowertrainData_11 ==
  GearNtrl_D_Stat : Constant
  GearNtrl_No_Cnt : Constant
  GearNtrl_No_Cs : Constant
  bus_creator : BusCreator  Inputs=3
  port : Outport
  wires:
  bus_creator/1 -> port/1  "PowertrainData_11"
  GearNtrl_D_Stat/1 -> bus_creator/1  "GearNtrl_D_Stat"
  GearNtrl_No_Cnt/1 -> bus_creator/2  "GearNtrl_No_Cnt"
  GearNtrl_No_Cs/1 -> bus_creator/3  "GearNtrl_No_Cs"

== system test_mdl/FD1_CAN_P702_GASD_MY21_DCV_V06/ECM_Diesel/PowertrainData_12 ==
  PtIgnSwtch_D_Stat : Constant
  PtIgnSwtch_No_Cnt : Constant
  PtIgnSwtch_No_Cs : Constant
  bus_creator : BusCreator  Inputs=3
  port : Outport
  wires:
  bus_creator/1 -> port/1  "PowertrainData_12"
  PtIgnSwtch_D_Stat/1 -> bus_creator/1  "PtIgnSwtch_D_Stat"
  PtIgnSwtch_No_Cnt/1 -> bus_creator/2  "PtIgnSwtch_No_Cnt"
  PtIgnSwtch_No_Cs/1 -> bus_creator/3  "PtIgnSwtch_No_Cs"

== system test_mdl/FD1_CAN_P702_GASD_MY21_DCV_V06/ECM_Diesel/PowertrainData_2 ==
  ApedPos_Pc_ActlDiag : Constant
  EngAirIn_Te_Actl : Constant
  EngClnt_Te_ActlDiag : Constant
  EngLoad_Pc_CalcDiag : Constant
  EngMsgTxt_D_Rq : Constant
  GrllShtrPos_B_Falt : Constant
  GrllShtrPos_D_Cmd : Constant
  IsaOffst_D_Stat : Constant
  ObdWarmUp_B_Complt : Constant
  SlMde_D_RqDsply : Constant
  SlMde_D_Stat : Constant
  bus_creator : BusCreator  Inputs=11
  port : Outport
  wires:
  bus_creator/1 -> port/1  "PowertrainData_2"
  ApedPos_Pc_ActlDiag/1 -> bus_creator/1  "ApedPos_Pc_ActlDiag"
  EngAirIn_Te_Actl/1 -> bus_creator/2  "EngAirIn_Te_Actl"
  EngClnt_Te_ActlDiag/1 -> bus_creator/3  "EngClnt_Te_ActlDiag"
  EngLoad_Pc_CalcDiag/1 -> bus_creator/4  "EngLoad_Pc_CalcDiag"
  EngMsgTxt_D_Rq/1 -> bus_creator/5  "EngMsgTxt_D_Rq"
  GrllShtrPos_B_Falt/1 -> bus_creator/6  "GrllShtrPos_B_Falt"
  GrllShtrPos_D_Cmd/1 -> bus_creator/7  "GrllShtrPos_D_Cmd"
  IsaOffst_D_Stat/1 -> bus_creator/8  "IsaOffst_D_Stat"
  ObdWarmUp_B_Complt/1 -> bus_creator/9  "ObdWarmUp_B_Complt"
  SlMde_D_RqDsply/1 -> bus_creator/10  "SlMde_D_RqDsply"
  SlMde_D_Stat/1 -> bus_creator/11  "SlMde_D_Stat"

== system test_mdl/FD1_CAN_P702_GASD_MY21_DCV_V06/ECM_Diesel/PowertrainData_3 ==
  BattULoChrg_U_Cmd : Constant
  ElLoadCtl_D_Rq : Constant
  EngMnfld_P_Actl : Constant
  FuelPumpPwr_B_Rq : Constant
  bus_creator : BusCreator  Inputs=4
  port : Outport
  wires:
  bus_creator/1 -> port/1  "PowertrainData_3"
  BattULoChrg_U_Cmd/1 -> bus_creator/1  "BattULoChrg_U_Cmd"
  ElLoadCtl_D_Rq/1 -> bus_creator/2  "ElLoadCtl_D_Rq"
  EngMnfld_P_Actl/1 -> bus_creator/3  "EngMnfld_P_Actl"
  FuelPumpPwr_B_Rq/1 -> bus_creator/4  "FuelPumpPwr_B_Rq"

== system test_mdl/FD1_CAN_P702_GASD_MY21_DCV_V06/ECM_Diesel/PowertrainData_6 ==
  BrkTot_Tq_RqFapLc : Constant
  FapLc_B_Err : Constant
  TrnAin_Pc_RqDrv : Constant
  bus_creator : BusCreator  Inputs=3
  port : Outport
  wires:
  bus_creator/1 -> port/1  "PowertrainData_6"
  BrkTot_Tq_RqFapLc/1 -> bus_creator/1  "BrkTot_Tq_RqFapLc"
  FapLc_B_Err/1 -> bus_creator/2  "FapLc_B_Err"
  TrnAin_Pc_RqDrv/1 -> bus_creator/3  "TrnAin_Pc_RqDrv"

== system test_mdl/FD1_CAN_P702_GASD_MY21_DCV_V06/ECM_Diesel/PowertrainData_7 ==
  EcoCochA_Pc_Dsply : Constant
  EcoCochCrus_Pc_Dsply : Constant
  EcoCochDecel_Pc_Dsply : Constant
  EcoCochIdlFuel_Pc_Dsply : Constant
  EcoCochInstNeg_B_Dsply : Constant
  EcoCochInst_Pc_Dsply : Constant
  EcoCochShif_Pc_Dsply : Constant
  bus_creator : BusCreator  Inputs=7
  port : Outport
  wires:
  bus_creator/1 -> port/1  "PowertrainData_7"
  EcoCochA_Pc_Dsply/1 -> bus_creator/1  "EcoCochA_Pc_Dsply"
  EcoCochCrus_Pc_Dsply/1 -> bus_creator/2  "EcoCochCrus_Pc_Dsply"
  EcoCochDecel_Pc_Dsply/1 -> bus_creator/3  "EcoCochDecel_Pc_Dsply"
  EcoCochIdlFuel_Pc_Dsply/1 -> bus_creator/4  "EcoCochIdlFuel_Pc_Dsply"
  EcoCochInstNeg_B_Dsply/1 -> bus_creator/5  "EcoCochInstNeg_B_Dsply"
  EcoCochInst_Pc_Dsply/1 -> bus_creator/6  "EcoCochInst_Pc_Dsply"
  EcoCochShif_Pc_Dsply/1 -> bus_creator/7  "EcoCochShif_Pc_Dsply"

== system test_mdl/FD1_CAN_P702_GASD_MY21_DCV_V06/ECM_Diesel/PowertrainData_9 ==
  AutoTowActv_B_Stat : Constant
  AutoTowAllw_D_StatMnu : Constant
  EngExhMdeQuiet_D2_Stat : Constant
  GrossTrainWeight_M_Est : Constant
  HvacCmprLim_D_Stat : Constant
  TrailCtlPt_B_Falt : Constant
  Veh_V_DsplyTrailCtlSet : Constant
  WakeAlarm1_B_Typ : Constant
  WakeAlarm1_T_Rq : Constant
  bus_creator : BusCreator  Inputs=9
  port : Outport
  wires:
  bus_creator/1 -> port/1  "PowertrainData_9"
  AutoTowActv_B_Stat/1 -> bus_creator/1  "AutoTowActv_B_Stat"
  AutoTowAllw_D_StatMnu/1 -> bus_creator/2  "AutoTowAllw_D_StatMnu"
  EngExhMdeQuiet_D2_Stat/1 -> bus_creator/3  "EngExhMdeQuiet_D2_Stat"
  GrossTrainWeight_M_Est/1 -> bus_creator/4  "GrossTrainWeight_M_Est"
  HvacCmprLim_D_Stat/1 -> bus_creator/5  "HvacCmprLim_D_Stat"
  TrailCtlPt_B_Falt/1 -> bus_creator/6  "TrailCtlPt_B_Falt"
  Veh_V_DsplyTrailCtlSet/1 -> bus_creator/7  "Veh_V_DsplyTrailCtlSet"
  WakeAlarm1_B_Typ/1 -> bus_creator/8  "WakeAlarm1_B_Typ"
  WakeAlarm1_T_Rq/1 -> bus_creator/9  "WakeAlarm1_T_Rq"

== system test_mdl/FD1_CAN_P702_GASD_MY21_DCV_V06/ECM_Diesel/Powertrain_Data_4 ==
  BpedDrvMsgTxt_B_Dsply : Constant
  FuelLvlWarn_D_ActlEng : Constant
  FuelLvl_Pc_DsplyEng : Constant
  FuelRange_L_DsplyEng : Constant
  RearDiffOilTeWarn_B_Rq : Constant
  RearDiffOil_Te_Actl : Constant
  SelDrvMdePt_D_Stat : Constant
  bus_creator : BusCreator  Inputs=7
  port : Outport
  wires:
  bus_creator/1 -> port/1  "Powertrain_Data_4"
  BpedDrvMsgTxt_B_Dsply/1 -> bus_creator/1  "BpedDrvMsgTxt_B_Dsply"
  FuelLvlWarn_D_ActlEng/1 -> bus_creator/2  "FuelLvlWarn_D_ActlEng"
  FuelLvl_Pc_DsplyEng/1 -> bus_creator/3  "FuelLvl_Pc_DsplyEng"
  FuelRange_L_DsplyEng/1 -> bus_creator/4  "FuelRange_L_DsplyEng"
  RearDiffOilTeWarn_B_Rq/1 -> bus_creator/5  "RearDiffOilTeWarn_B_Rq"
  RearDiffOil_Te_Actl/1 -> bus_creator/6  "RearDiffOil_Te_Actl"
  SelDrvMdePt_D_Stat/1 -> bus_creator/7  "SelDrvMdePt_D_Stat"

== system test_mdl/FD1_CAN_P702_GASD_MY21_DCV_V06/ECM_Diesel/Powertrain_Data_5 ==
  AdasLcObtclAbrt_B_Stat : Constant
  AirDamPos_D_Stat : Constant
  BattRgenLoChrg_D_RqEng : Constant
  BattRgenLoDChrg_D_RqEng : Constant
  FapLcActv_B_Stat : Constant
  FapLcInhbt_B_Rq : Constant
  FapLcMaxGrdAbrt_B_Stat : Constant
  FapLcMaxGrdInhbt_B_Stat : Constant
  FapLcObstcl_B_Stat : Constant
  FapLcPrchgBrk_B_Rq : Constant
  FapLcStopHold_B_Rq : Constant
  bus_creator : BusCreator  Inputs=11
  port : Outport
  wires:
  bus_creator/1 -> port/1  "Powertrain_Data_5"
  AdasLcObtclAbrt_B_Stat/1 -> bus_creator/1  "AdasLcObtclAbrt_B_Stat"
  AirDamPos_D_Stat/1 -> bus_creator/2  "AirDamPos_D_Stat"
  BattRgenLoChrg_D_RqEng/1 -> bus_creator/3  "BattRgenLoChrg_D_RqEng"
  BattRgenLoDChrg_D_RqEng/1 -> bus_creator/4  "BattRgenLoDChrg_D_RqEng"
  FapLcActv_B_Stat/1 -> bus_creator/5  "FapLcActv_B_Stat"
  FapLcInhbt_B_Rq/1 -> bus_creator/6  "FapLcInhbt_B_Rq"
  FapLcMaxGrdAbrt_B_Stat/1 -> bus_creator/7  "FapLcMaxGrdAbrt_B_Stat"
  FapLcMaxGrdInhbt_B_Stat/1 -> bus_creator/8  "FapLcMaxGrdInhbt_B_Stat"
  FapLcObstcl_B_Stat/1 -> bus_creator/9  "FapLcObstcl_B_Stat"
  FapLcPrchgBrk_B_Rq/1 -> bus_creator/10  "FapLcPrchgBrk_B_Rq"
  FapLcStopHold_B_Rq/1 -> bus_creator/11  "FapLcStopHold_B_Rq"

== system test_mdl/FD1_CAN_P702_GASD_MY21_DCV_V06/ECM_Diesel/Stop_Start ==
  AutoStopPtDelta_I_Est : Constant
  HiElPwInhbt_B_Stat : Constant
  OdoTripVerify_L_Actl : Constant
  StopStrtDrvMde_D_Indic : Constant
  StopStrtIODTxt_D_Rq : Constant
  StopStrtMsgTxt_D_Rq : Constant
  StopStrtStdby_D_Indic : Constant
  bus_creator : BusCreator  Inputs=7
  port : Outport
  wires:
  bus_creator/1 -> port/1  "Stop_Start"
  AutoStopPtDelta_I_Est/1 -> bus_creator/1  "AutoStopPtDelta_I_Est"
  HiElPwInhbt_B_Stat/1 -> bus_creator/2  "HiElPwInhbt_B_Stat"
  OdoTripVerify_L_Actl/1 -> bus_creator/3  "OdoTripVerify_L_Actl"
  StopStrtDrvMde_D_Indic/1 -> bus_creator/4  "StopStrtDrvMde_D_Indic"
  StopStrtIODTxt_D_Rq/1 -> bus_creator/5  "StopStrtIODTxt_D_Rq"
  StopStrtMsgTxt_D_Rq/1 -> bus_creator/6  "StopStrtMsgTxt_D_Rq"
  StopStrtStdby_D_Indic/1 -> bus_creator/7  "StopStrtStdby_D_Indic"

== system test_mdl/FD1_CAN_P702_GASD_MY21_DCV_V06/ECM_Diesel/TesterPhysicalResPCM ==
  TesterPhysicalResPCM : Constant
  bus_creator : BusCreator  Inputs=1
  port : Outport
  wires:
  bus_creator/1 -> port/1  "TesterPhysicalResPCM"
  TesterPhysicalResPCM/1 -> bus_creator/1  "TesterPhysicalResPCM"

== system test_mdl/FD1_CAN_P702_GASD_MY21_DCV_V06/ECM_Diesel/TesterPhysicalResSOBDMCFD1 ==
  TesterPhysicalResSOBDMC : Constant
  bus_creator : BusCreator  Inputs=1
  port : Outport
  wires:
  bus_creator/1 -> port/1  "TesterPhysicalResSOBDMCFD1"
  TesterPhysicalResSOBDMC/1 -> bus_creator/1  "TesterPhysicalResSOBDMC"

== system test_mdl/FD1_CAN_P702_GASD_MY21_DCV_V06/ECM_Diesel/TorqueDataEngFlags ==
  PrplWhlTotTqRq_No_Cnt : Constant
  PrplWhlTotTqRq_No_Cs : Constant
  PrplWhlTot_Tq_LimMn : Constant
  PrplWhlTot_Tq_Rq : Constant
  PtDrvMde_D_Stat : Constant
  bus_creator : BusCreator  Inputs=5
  port : Outport
  wires:
  bus_creator/1 -> port/1  "TorqueDataEngFlags"
  PrplWhlTotTqRq_No_Cnt/1 -> bus_creator/1  "PrplWhlTotTqRq_No_Cnt"
  PrplWhlTotTqRq_No_Cs/1 -> bus_creator/2  "PrplWhlTotTqRq_No_Cs"
  PrplWhlTot_Tq_LimMn/1 -> bus_creator/3  "PrplWhlTot_Tq_LimMn"
  PrplWhlTot_Tq_Rq/1 -> bus_creator/4  "PrplWhlTot_Tq_Rq"
  PtDrvMde_D_Stat/1 -> bus_creator/5  "PtDrvMde_D_Stat"

== system test_mdl/FD1_CAN_P702_GASD_MY21_DCV_V06/ECM_Diesel/VehicleOperatingModes ==
  ElPw_D_Stat : Constant
  ElPw_D_StatStrtStop : Constant
  Eng_D_Stat : Constant
  PlgActvArb_B_Actl : Constant
  PrplWhlRgenMn_Tq_Actl : Constant
  PrplWhlTot2_Tq_Actl : Constant
  PwPckTq_D_Stat : Constant
  TrnAinTq_D_Qf : Constant
  TrnAin_Tq_Actl : Constant
  bus_creator : BusCreator  Inputs=9
  port : Outport
  wires:
  bus_creator/1 -> port/1  "VehicleOperatingModes"
  ElPw_D_Stat/1 -> bus_creator/1  "ElPw_D_Stat"
  ElPw_D_StatStrtStop/1 -> bus_creator/2  "ElPw_D_StatStrtStop"
  Eng_D_Stat/1 -> bus_creator/3  "Eng_D_Stat"
  PlgActvArb_B_Actl/1 -> bus_creator/4  "PlgActvArb_B_Actl"
  PrplWhlRgenMn_Tq_Actl/1 -> bus_creator/5  "PrplWhlRgenMn_Tq_Actl"
  PrplWhlTot2_Tq_Actl/1 -> bus_creator/6  "PrplWhlTot2_Tq_Actl"
  PwPckTq_D_Stat/1 -> bus_creator/7  "PwPckTq_D_Stat"
  TrnAinTq_D_Qf/1 -> bus_creator/8  "TrnAinTq_D_Qf"
  TrnAin_Tq_Actl/1 -> bus_creator/9  "TrnAin_Tq_Actl"
